simulink subsystem "encoderOld"  (R2020b)
settings: Solver=VariableStepAuto  StartTime=0.0  StopTime=10.0  RelTol=1e-3
settings Model: Creator=LeonK  LastModifiedBy=LeonK
settings DebuggingCC: UnconnectedInputMsg=none  UnconnectedOutputMsg=none  UnconnectedLineMsg=none  SFMachineParentedDataDiag=error
settings ModelReferenceCC: EnableRefExpFcnMdlSchedulingChecks=off

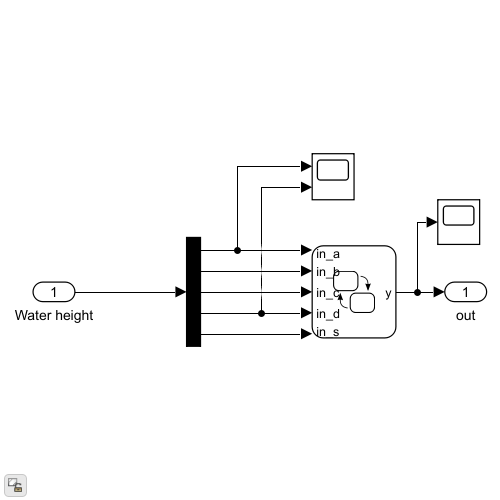
[thumbnail: Simulink's stored preview of the top-level diagram]
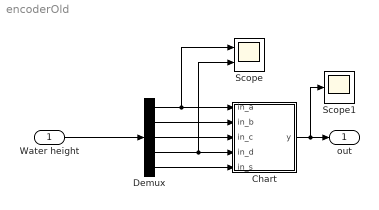
== system encoderOld ==
  Water height : Inport
  Chart : Stateflow chart  TreatAsAtomicUnit=on
  Demux : Demux  Outputs=5
  Scope : Scope  NumInputPorts=2
  Scope1 : Scope
  out : Outport
  wires:
  Demux/1 -> Chart/1(in_a), Scope/1
  Demux/2 -> Chart/2(in_b)
  Demux/3 -> Chart/3(in_c)
  Demux/4 -> Chart/4(in_d), Scope/2
  Chart/1(y) -> out/1, Scope1/1
  Water height/1 -> Demux/1
  Demux/5 -> Chart/5(in_s)

== stateflow chart encoderOld/Chart ==
  state q_initialize
  state q0
  state q_0_10
  state q_10_20
  state q_20_30
  state q_30_max
  state flooding
  state q_malfunction
  q_initialize -> q_30_max [order 2] : [in_a==1]{y=1}
  q_10_20 -> q_10_20 [order 4] : [in_c==1]{y=-1;}
  q_20_30 -> q_20_30 [order 4] : [in_b==1]{y=-1;}
  q_0_10 -> q_10_20 [order 1] : [in_c==1]{y=1;}
  (default) -> q_initialize
  q0 -> q_0_10 [order 2] : [in_d==1]{y=1;}
  q_initialize -> q0 [order 1] : [in_a==0]{y=0;}
  q_10_20 -> q_20_30 [order 2] : [in_b==1]{y=1;}
  q_20_30 -> q_30_max [order 2] : [in_a==1]{y=1;}
  q_30_max -> q_30_max [order 4] : [in_a==1]{y=-1;}
  q_30_max -> flooding [order 3] : [in_s==1]{y=1;y=1;y=1;y=1;y=1;}
  q0 -> q0 [order 1] : [in_d==0]{y=-1;}
  q_0_10 -> q0 [order 2] : [in_d==0]{y=0;}
  q_0_10 -> q_0_10 [order 3] : [in_d==1]{y=-1;}
  q_10_20 -> q_0_10 [order 3] : [in_c==0]{y=0;}
  q_10_20 -> q_malfunction [order 1] : [in_d==0]{y=0;y=0;y=0;y=0;y=0;}
  q_20_30 -> q_malfunction [order 1] : [in_d==0||in_c==0]{y=0;y=0;y=0;y=0;y=0;}
  q_30_max -> q_malfunction [order 1] : [in_d==0||in_c==0||in_b==0]{y=0;y=0;y=0;y=0;y=0;}
  q_20_30 -> q_10_20 [order 3] : [in_b==0]{y=0;}
  q_30_max -> q_20_30 [order 2] : [in_a==0]{y=0;}
  data: in_a input; in_b input; in_c input; in_d input; in_s input; y output
